simulink model "String1_Diode_P"  (R2023b)
settings: Solver=VariableStepAuto  StartTime=0.0  StopTime=10.0  RelTol=1e-3
undefined symbols (not defined in the file or in its folder): Slope_Vdc_string1
libraries: SolarCellLibrary x23, spsCurrentMeasurementLib x1, spsControlledVoltageSourceLib x1, simulink x1, spsVoltageMeasurementLib x1
settings Model: Creator=kevin  LastModifiedBy=kevin

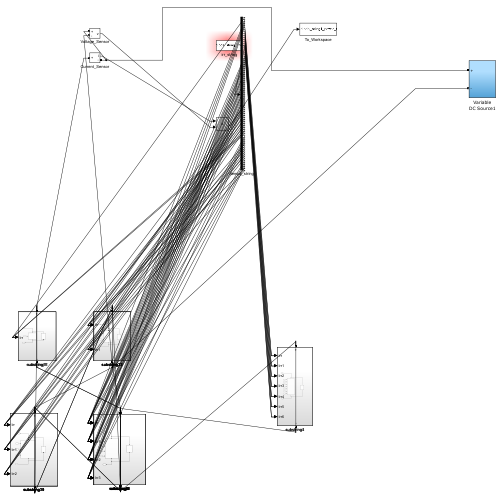
[thumbnail: Simulink's stored preview of the top-level diagram]
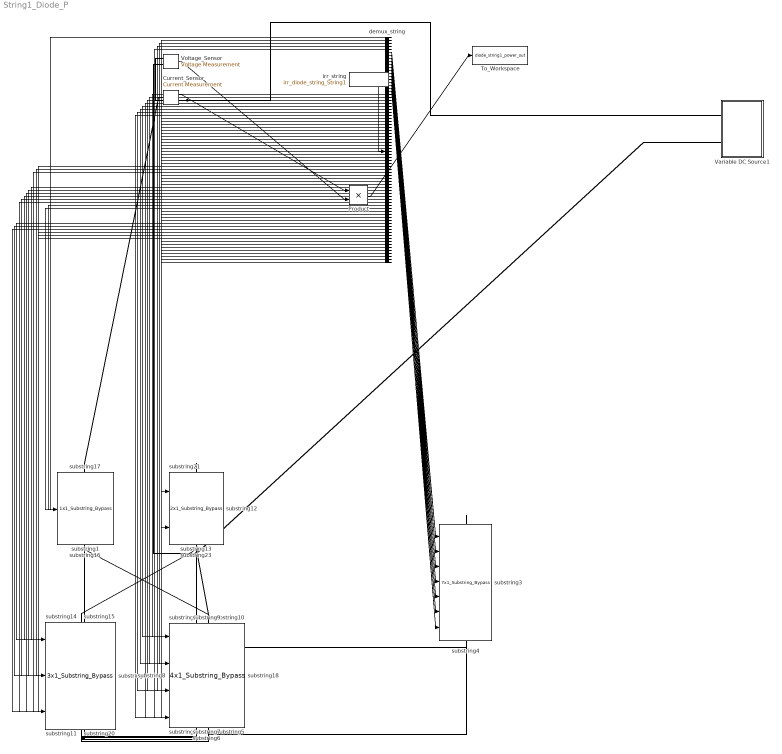
== system String1_Diode_P ==
  Current_Sensor : spsCurrentMeasurementLib/Current Measurement  PhasorSimulation=off  OutputType=Complex  PSBequivalent=0
  Product : Product
  To_Workspace : ToWorkspace  VariableName=diode_string1_power_out  SaveFormat=Timeseries  SampleTime=-1
  Variable DC Source1 : Subsystem
  Voltage_Sensor : spsVoltageMeasurementLib/Voltage Measurement  PhasorSimulation=off  OutputType=Complex  PSBequivalent=0
  demux_string : Demux  Outputs=76
  irr_string : FromWorkspace  VariableName=irr_diode_string_String1
  substring1 : SolarCellLibrary/1x1_Substring_Bypass  SystemSampleTime=-1  VariantActivationTime=update diagram  AllowFlexibleInterface=on  Latency=0  AutoFrameSizeCalculation=off
      settings: PortSchema="{\"entries\":[{\"content\":{\"sides\":[{\"content\":{\"connectorIds\":[\"In1\"]},\"type\":\"ConnectorPlacement.EquallySpacedRectSide\",\"uuid\":\"016f4cc6-4ebe-4f80-ac8d-7f3fb38a55cf\"},{\"content\":{\"side\":\"RIGHT\"},\"type\":\"ConnectorPlacement.EquallySpacedRectSide\",\"uuid\":\"d11369f5-d005-4384-9051-e7de8060ac42\"},{\"content\":{\"connectorIds\":[\"LConn1\"],\"side\":\"TOP\"},\"type\":\"ConnectorPlacement.EquallySpacedRectSide\",\"uuid\":\"3f2fb0fa-159f-4323-a4c6-2fcef805006a\"},{\"content\":{\"connectorIds\":[\"RConn1\"],\"side\":\"BOTTOM\"},\"type\":\"ConnectorPlacement.EquallySpacedRectSide\",\"uuid\":\"9614dff7-9527-41d7-b7c0-8c4e335b1ea1\"}]},\"type\":\"ConnectorPlacement.EquallySpacedConnector\",\"uuid\":\"053d9fdb-3f20-4ed6-b8eb-465c401ad454\"}],\"packageUris\":[\"http://schema.mathworks.com/mf0/Connector/R2020b\"],\"version\":\"1.0\"}"
  substring{2,5..10,18,22} (9 alike) : SolarCellLibrary/4x1_Substring_Bypass  SystemSampleTime=-1  VariantActivationTime=update diagram  AllowFlexibleInterface=on  Latency=0  AutoFrameSizeCalculation=off
      settings: PortSchema="{\"entries\":[{\"content\":{\"sides\":[{\"content\":{\"connectorIds\":[\"In1\",\"In2\",\"In3\",\"In4\"]},\"type\":\"ConnectorPlacement.EquallySpacedRectSide\",\"uuid\":\"0ad94482-327f-42a8-a753-929b8c21c598\"},{\"content\":{\"side\":\"RIGHT\"},\"type\":\"ConnectorPlacement.EquallySpacedRectSide\",\"uuid\":\"447f9d08-5865-4684-a5c5-74ffbb93afc8\"},{\"content\":{\"connectorIds\":[\"LConn1\"],\"side\":\"TOP\"},\"type\":\"ConnectorPlacement.EquallySpacedRectSide\",\"uuid\":\"4f0b0805-593f-452f-8bf0-062e33ae5583\"},{\"content\":{\"connectorIds\":[\"RConn1\"],\"side\":\"BOTTOM\"},\"type\":\"ConnectorPlacement.EquallySpacedRectSide\",\"uuid\":\"b069b9dc-d744-4b07-9d86-0222f837bdcc\"}]},\"type\":\"ConnectorPlacement.EquallySpacedConnector\",\"uuid\":\"0517c35b-d064-4567-8e0e-3ac38b35b549\"}],\"packageUris\":[\"http://schema.mathworks.com/mf0/Connector/R2020b\"],\"version\":\"1.0\"}"
  substring{11,14..15,19..20} (5 alike) : SolarCellLibrary/3x1_Substring_Bypass  SystemSampleTime=-1  VariantActivationTime=update diagram  AllowFlexibleInterface=on  Latency=0  AutoFrameSizeCalculation=off
      settings: PortSchema="{\"entries\":[{\"content\":{\"sides\":[{\"content\":{\"connectorIds\":[\"In1\",\"In2\",\"In3\"]},\"type\":\"ConnectorPlacement.EquallySpacedRectSide\",\"uuid\":\"e1573c16-3472-4da1-87e4-7e9113dfd0da\"},{\"content\":{\"side\":\"RIGHT\"},\"type\":\"ConnectorPlacement.EquallySpacedRectSide\",\"uuid\":\"6d8234c9-0139-42ab-bb54-774f3f086f97\"},{\"content\":{\"connectorIds\":[\"LConn1\"],\"side\":\"TOP\"},\"type\":\"ConnectorPlacement.EquallySpacedRectSide\",\"uuid\":\"060201bf-918d-4a08-b0b9-041cda264031\"},{\"content\":{\"connectorIds\":[\"RConn1\"],\"side\":\"BOTTOM\"},\"type\":\"ConnectorPlacement.EquallySpacedRectSide\",\"uuid\":\"1d8121d5-0537-4208-a815-529662f49494\"}]},\"type\":\"ConnectorPlacement.EquallySpacedConnector\",\"uuid\":\"44fb3434-6009-4cd2-b602-382939d4eccc\"}],\"packageUris\":[\"http://schema.mathworks.com/mf0/Connector/R2020b\"],\"version\":\"1.0\"}"
  substring{12..13,21,23} (4 alike) : SolarCellLibrary/2x1_Substring_Bypass  SystemSampleTime=-1  VariantActivationTime=update diagram  AllowFlexibleInterface=on  Latency=0  AutoFrameSizeCalculation=off
      settings: PortSchema="{\"entries\":[{\"content\":{\"sides\":[{\"content\":{\"connectorIds\":[\"In1\",\"In2\"]},\"type\":\"ConnectorPlacement.EquallySpacedRectSide\",\"uuid\":\"a5963537-3d0a-4548-96d6-ee15d8c928e2\"},{\"content\":{\"side\":\"RIGHT\"},\"type\":\"ConnectorPlacement.EquallySpacedRectSide\",\"uuid\":\"05aa206f-a774-4b6c-88a9-60bc940310ec\"},{\"content\":{\"connectorIds\":[\"LConn1\"],\"side\":\"TOP\"},\"type\":\"ConnectorPlacement.EquallySpacedRectSide\",\"uuid\":\"4b4ddc51-41e7-4a03-b4ed-22494227b586\"},{\"content\":{\"connectorIds\":[\"RConn1\"],\"side\":\"BOTTOM\"},\"type\":\"ConnectorPlacement.EquallySpacedRectSide\",\"uuid\":\"2c9efdb8-7817-4fe0-aba5-e8b0ca6dcca8\"}]},\"type\":\"ConnectorPlacement.EquallySpacedConnector\",\"uuid\":\"ce0bb1d9-3157-48c9-8260-965824e28996\"}],\"packageUris\":[\"http://schema.mathworks.com/mf0/Connector/R2020b\"],\"version\":\"1.0\"}"
  substring16 : SolarCellLibrary/1x1_Substring_Bypass  SystemSampleTime=-1  VariantActivationTime=update diagram  AllowFlexibleInterface=on  Latency=0  AutoFrameSizeCalculation=off
      settings: PortSchema="{\"entries\":[{\"content\":{\"sides\":[{\"content\":{\"connectorIds\":[\"In1\"]},\"type\":\"ConnectorPlacement.EquallySpacedRectSide\",\"uuid\":\"016f4cc6-4ebe-4f80-ac8d-7f3fb38a55cf\"},{\"content\":{\"side\":\"RIGHT\"},\"type\":\"ConnectorPlacement.EquallySpacedRectSide\",\"uuid\":\"d11369f5-d005-4384-9051-e7de8060ac42\"},{\"content\":{\"connectorIds\":[\"LConn1\"],\"side\":\"TOP\"},\"type\":\"ConnectorPlacement.EquallySpacedRectSide\",\"uuid\":\"3f2fb0fa-159f-4323-a4c6-2fcef805006a\"},{\"content\":{\"connectorIds\":[\"RConn1\"],\"side\":\"BOTTOM\"},\"type\":\"ConnectorPlacement.EquallySpacedRectSide\",\"uuid\":\"9614dff7-9527-41d7-b7c0-8c4e335b1ea1\"}]},\"type\":\"ConnectorPlacement.EquallySpacedConnector\",\"uuid\":\"053d9fdb-3f20-4ed6-b8eb-465c401ad454\"}],\"packageUris\":[\"http://schema.mathworks.com/mf0/Connector/R2020b\"],\"version\":\"1.0\"}"
  substring17 : SolarCellLibrary/1x1_Substring_Bypass  SystemSampleTime=-1  VariantActivationTime=update diagram  AllowFlexibleInterface=on  Latency=0  AutoFrameSizeCalculation=off
      settings: PortSchema="{\"entries\":[{\"content\":{\"sides\":[{\"content\":{\"connectorIds\":[\"In1\"]},\"type\":\"ConnectorPlacement.EquallySpacedRectSide\",\"uuid\":\"016f4cc6-4ebe-4f80-ac8d-7f3fb38a55cf\"},{\"content\":{\"side\":\"RIGHT\"},\"type\":\"ConnectorPlacement.EquallySpacedRectSide\",\"uuid\":\"d11369f5-d005-4384-9051-e7de8060ac42\"},{\"content\":{\"connectorIds\":[\"LConn1\"],\"side\":\"TOP\"},\"type\":\"ConnectorPlacement.EquallySpacedRectSide\",\"uuid\":\"3f2fb0fa-159f-4323-a4c6-2fcef805006a\"},{\"content\":{\"connectorIds\":[\"RConn1\"],\"side\":\"BOTTOM\"},\"type\":\"ConnectorPlacement.EquallySpacedRectSide\",\"uuid\":\"9614dff7-9527-41d7-b7c0-8c4e335b1ea1\"}]},\"type\":\"ConnectorPlacement.EquallySpacedConnector\",\"uuid\":\"053d9fdb-3f20-4ed6-b8eb-465c401ad454\"}],\"packageUris\":[\"http://schema.mathworks.com/mf0/Connector/R2020b\"],\"version\":\"1.0\"}"
  substring3 : SolarCellLibrary/7x1_Substring_Bypass  SystemSampleTime=-1  VariantActivationTime=update diagram  AllowFlexibleInterface=on  Latency=0  AutoFrameSizeCalculation=off
      settings: PortSchema="{\"entries\":[{\"content\":{\"sides\":[{\"content\":{\"connectorIds\":[\"In1\",\"In2\",\"In3\",\"In4\",\"In5\",\"In6\",\"In7\"]},\"type\":\"ConnectorPlacement.EquallySpacedRectSide\",\"uuid\":\"c5d06187-c1e0-4d91-835c-ee29588cb44f\"},{\"content\":{\"side\":\"RIGHT\"},\"type\":\"ConnectorPlacement.EquallySpacedRectSide\",\"uuid\":\"fd9f7d20-5ecf-46c9-863a-3a3547d8be6c\"},{\"content\":{\"connectorIds\":[\"LConn1\"],\"side\":\"TOP\"},\"type\":\"ConnectorPlacement.EquallySpacedRectSide\",\"uuid\":\"062659ca-a252-445c-9ccd-4da921a84b50\"},{\"content\":{\"connectorIds\":[\"RConn1\"],\"side\":\"BOTTOM\"},\"type\":\"ConnectorPlacement.EquallySpacedRectSide\",\"uuid\":\"c76e3d95-a283-4347-bd23-f517150f3280\"}]},\"type\":\"ConnectorPlacement.EquallySpacedConnector\",\"uuid\":\"40a737f5-b71b-4c56-a946-02f4df997521\"}],\"packageUris\":[\"http://schema.mathworks.com/mf0/Connector/R2020b\"],\"version\":\"1.0\"}"
  substring4 : SolarCellLibrary/7x1_Substring_Bypass  SystemSampleTime=-1  VariantActivationTime=update diagram  AllowFlexibleInterface=on  Latency=0  AutoFrameSizeCalculation=off
      settings: PortSchema="{\"entries\":[{\"content\":{\"sides\":[{\"content\":{\"connectorIds\":[\"In1\",\"In2\",\"In3\",\"In4\",\"In5\",\"In6\",\"In7\"]},\"type\":\"ConnectorPlacement.EquallySpacedRectSide\",\"uuid\":\"c5d06187-c1e0-4d91-835c-ee29588cb44f\"},{\"content\":{\"side\":\"RIGHT\"},\"type\":\"ConnectorPlacement.EquallySpacedRectSide\",\"uuid\":\"fd9f7d20-5ecf-46c9-863a-3a3547d8be6c\"},{\"content\":{\"connectorIds\":[\"LConn1\"],\"side\":\"TOP\"},\"type\":\"ConnectorPlacement.EquallySpacedRectSide\",\"uuid\":\"062659ca-a252-445c-9ccd-4da921a84b50\"},{\"content\":{\"connectorIds\":[\"RConn1\"],\"side\":\"BOTTOM\"},\"type\":\"ConnectorPlacement.EquallySpacedRectSide\",\"uuid\":\"c76e3d95-a283-4347-bd23-f517150f3280\"}]},\"type\":\"ConnectorPlacement.EquallySpacedConnector\",\"uuid\":\"40a737f5-b71b-4c56-a946-02f4df997521\"}],\"packageUris\":[\"http://schema.mathworks.com/mf0/Connector/R2020b\"],\"version\":\"1.0\"}"
  wires:
  irr_string/1 -> demux_string/1
  demux_string/1 -> substring1/1
  demux_string/2 -> substring2/1
  demux_string/3 -> substring2/2
  demux_string/4 -> substring2/3
  demux_string/5 -> substring2/4
  demux_string/6 -> substring3/1
  demux_string/7 -> substring3/2
  demux_string/8 -> substring3/3
  demux_string/9 -> substring3/4
  demux_string/10 -> substring3/5
  demux_string/11 -> substring3/6
  demux_string/12 -> substring3/7
  demux_string/13 -> substring4/1
  demux_string/14 -> substring4/2
  demux_string/15 -> substring4/3
  demux_string/16 -> substring4/4
  demux_string/17 -> substring4/5
  demux_string/18 -> substring4/6
  demux_string/19 -> substring4/7
  demux_string/20 -> substring5/1
  demux_string/21 -> substring5/2
  demux_string/22 -> substring5/3
  demux_string/23 -> substring5/4
  demux_string/24 -> substring6/1
  demux_string/25 -> substring6/2
  demux_string/26 -> substring6/3
  demux_string/27 -> substring6/4
  demux_string/28 -> substring7/1
  demux_string/29 -> substring7/2
  demux_string/30 -> substring7/3
  demux_string/31 -> substring7/4
  demux_string/32 -> substring8/1
  demux_string/33 -> substring8/2
  demux_string/34 -> substring8/3
  demux_string/35 -> substring8/4
  demux_string/36 -> substring9/1
  demux_string/37 -> substring9/2
  demux_string/38 -> substring9/3
  demux_string/39 -> substring9/4
  demux_string/40 -> substring10/1
  demux_string/41 -> substring10/2
  demux_string/42 -> substring10/3
  demux_string/43 -> substring10/4
  demux_string/44 -> substring11/1
  demux_string/45 -> substring11/2
  demux_string/46 -> substring11/3
  demux_string/47 -> substring12/1
  demux_string/48 -> substring12/2
  demux_string/49 -> substring13/1
  demux_string/50 -> substring13/2
  demux_string/51 -> substring14/1
  demux_string/52 -> substring14/2
  demux_string/53 -> substring14/3
  demux_string/54 -> substring15/1
  demux_string/55 -> substring15/2
  demux_string/56 -> substring15/3
  demux_string/57 -> substring16/1
  demux_string/58 -> substring17/1
  demux_string/59 -> substring18/1
  demux_string/60 -> substring18/2
  demux_string/61 -> substring18/3
  demux_string/62 -> substring18/4
  demux_string/63 -> substring19/1
  demux_string/64 -> substring19/2
  demux_string/65 -> substring19/3
  demux_string/66 -> substring20/1
  demux_string/67 -> substring20/2
  demux_string/68 -> substring20/3
  demux_string/69 -> substring21/1
  demux_string/70 -> substring21/2
  demux_string/71 -> substring22/1
  demux_string/72 -> substring22/2
  demux_string/73 -> substring22/3
  demux_string/74 -> substring22/4
  demux_string/75 -> substring23/1
  demux_string/76 -> substring23/2
  Current_Sensor/1 -> Product/1
  Voltage_Sensor/1 -> Product/2
  Product/1 -> To_Workspace/1
  connections:
  substring2/LConn1 -- substring1/RConn1
  substring3/LConn1 -- substring2/RConn1
  substring4/LConn1 -- substring3/RConn1
  substring5/LConn1 -- substring4/RConn1
  substring6/LConn1 -- substring5/RConn1
  substring7/LConn1 -- substring6/RConn1
  substring8/LConn1 -- substring7/RConn1
  substring9/LConn1 -- substring8/RConn1
  substring10/LConn1 -- substring9/RConn1
  substring11/LConn1 -- substring10/RConn1
  substring12/LConn1 -- substring11/RConn1
  substring13/LConn1 -- substring12/RConn1
  substring14/LConn1 -- substring13/RConn1
  substring15/LConn1 -- substring14/RConn1
  substring16/LConn1 -- substring15/RConn1
  substring17/LConn1 -- substring16/RConn1
  substring18/LConn1 -- substring17/RConn1
  substring19/LConn1 -- substring18/RConn1
  substring20/LConn1 -- substring19/RConn1
  substring21/LConn1 -- substring20/RConn1
  substring22/LConn1 -- substring21/RConn1
  substring23/LConn1 -- substring22/RConn1
  substring1/LConn1 -- Current_Sensor/LConn1
  Current_Sensor/RConn1 -- Variable DC Source1/LConn1 -- Voltage_Sensor/LConn1
  substring23/RConn1 -- Variable DC Source1/LConn2 -- Voltage_Sensor/LConn2

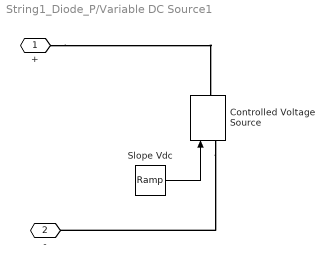
== system String1_Diode_P/Variable DC Source1 ==
  Controlled Voltage Source : spsControlledVoltageSourceLib/Controlled Voltage Source  Initialize=on  Source_Type=DC  Amplitude=0  Phase=0  Frequency=0  Measurements=None
  Slope Vdc : simulink/Sources/Ramp  slope=Slope_Vdc_string1  start=0  InitialOutput=0
  + : PMIOPort  Side=Left
  - : PMIOPort  Port=2  Side=Left
  wires:
  Slope Vdc/1 -> Controlled Voltage Source/1
  connections:
  Controlled Voltage Source/LConn1 -- -/RConn1
  +/RConn1 -- Controlled Voltage Source/RConn1
